simulink model "TH_P_Inv"  (R2023a)
settings: Solver=ode23  StartTime=0.0  StopTime=0.1  RelTol=1e-3
libraries: spsIGBTDiodeLib x6, simulink x3, spsSeriesRLCBranchLib x3, spsDCVoltageSourceLib x1, spsGroundLib x1, spsThreePhaseVIMeasurementLib x1, sps_lib x1

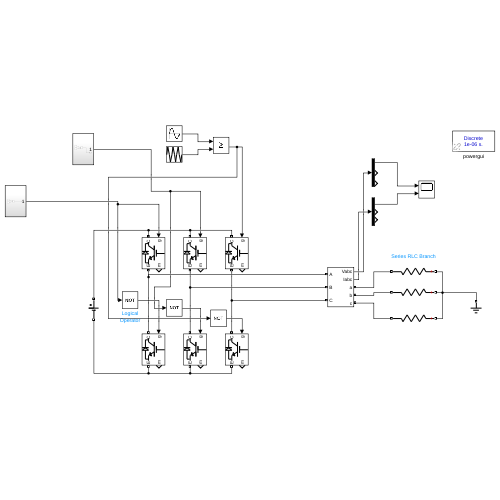
[thumbnail: Simulink's stored preview of the top-level diagram]
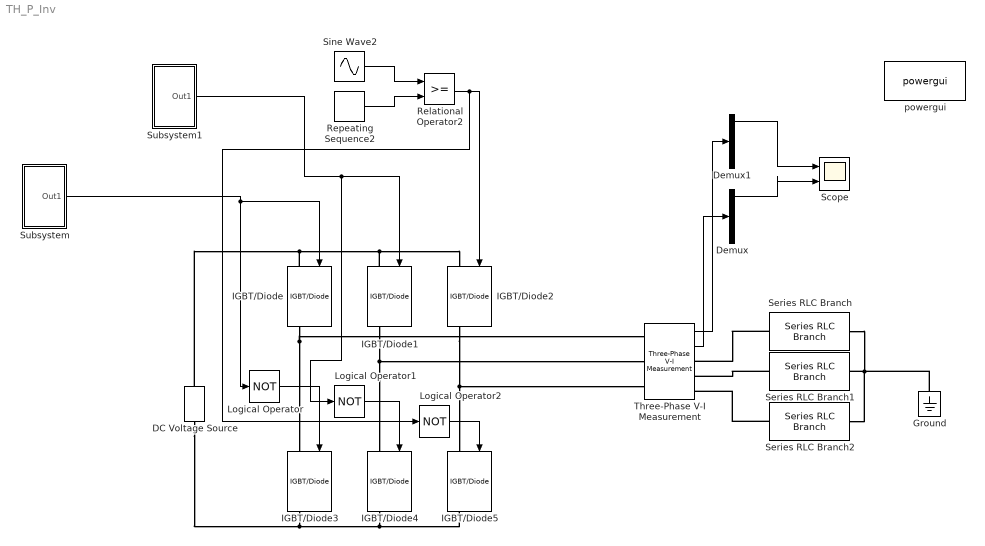
== system TH_P_Inv ==
  DC Voltage Source : spsDCVoltageSourceLib/DC Voltage Source  Amplitude=650  Measurements=None
  Demux : Demux  Outputs=3
  Demux1 : Demux  Outputs=3
  Ground : spsGroundLib/Ground  LConnTagsString=a
  IGBT/Diode{,1..5} (6 alike) : spsIGBTDiodeLib/IGBT//Diode  Ron=1e-3  Rs=1e5  Cs=inf  Measurements=on
  Logical Operator : Logic  Operator=NOT  AllPortsSameDT=off  OutDataTypeStr=boolean
  Logical Operator1 : Logic  Operator=NOT  AllPortsSameDT=off  OutDataTypeStr=boolean
  Logical Operator2 : Logic  Operator=NOT  AllPortsSameDT=off  OutDataTypeStr=boolean
  Relational Operator2 : RelationalOperator  OutDataTypeStr=boolean  RndMeth=Simplest  InputSameDT=off
  Repeating Sequence2 : simulink/Sources/Repeating Sequence  rep_seq_t=[0 0.25/5000 0.5/5000 0.75/5000 1/5000]  rep_seq_y=[0 1 0 -1 0 ]
  Scope : Scope  NumInputPorts=2
  Series RLC Branch : spsSeriesRLCBranchLib/Series RLC Branch  LConnTagsString=__new0  RConnTagsString=__new0  BranchType=R  Resistance=10  Inductance=1e-3  SetiL0=off  InitialCurrent=0  Capacitance=1e-6  Setx0=off  InitialVoltage=0  Measurements=None
  Series RLC Branch1 : spsSeriesRLCBranchLib/Series RLC Branch  LConnTagsString=__new0  RConnTagsString=__new0  BranchType=R  Resistance=10  Inductance=1e-3  SetiL0=off  InitialCurrent=0  Capacitance=1e-6  Setx0=off  InitialVoltage=0  Measurements=None
  Series RLC Branch2 : spsSeriesRLCBranchLib/Series RLC Branch  LConnTagsString=__new0  RConnTagsString=__new0  BranchType=R  Resistance=10  Inductance=1e-3  SetiL0=off  InitialCurrent=0  Capacitance=1e-6  Setx0=off  InitialVoltage=0  Measurements=None
  Sine Wave2 : Sin  Amplitude=0.99  Frequency=100*pi  Phase=(4*pi)/3  SampleTime=0
  Subsystem : Subsystem
  Subsystem1 : Subsystem
  Three-Phase V-I Measurement : spsThreePhaseVIMeasurementLib/Three-Phase V-I Measurement  VoltageMeasurement=phase-to-ground  SetLabelV=off  LabelV=Vabc  Vpu=off  VpuLL=off  CurrentMeasurement=yes  SetLabelI=off  LabelI=Iabc  Ipu=off  Pbase=100e6  Vbase=500e3  OutputType=Complex  PhasorSimulation=off  PSBequivalent=0
  powergui : sps_lib/powergui  Priority=1  SimulationMode=Discrete  SampleTime=1e-6  frequency=60  Iterations=50  frequencyindice=0  Pbase=100e6  ErrMax=1e-4  UnitsV=kV  UnitsW=MW  buscounter=0  FunctionMessages=off  echomessages=off  EnableUseOfTLC=off  CurrentSourceSwitches=off  DisableSnubberDevices=off  DisableRonSwitches=off  DisableVfSwitches=off  DisplayEquations=off  AutomaticDiscreteSolvers=off  SolverType=Tustin/Backward Euler (TBE)  Interpol=off  ExternalGateDelay=off  methode=off  Ts=100  x0status=blocks  SPID=on  SwTol=0  HookPort=off  NonlinearTolerance=1e-4  nMaxIteration=100  ContinueOnMaxIteration=off  RestoreLinks=warning  ResistiveCurrentMeasurement=off  Frange=[0:2:500]  Ylog=off  Xlog=on  ShowGrid=off  save=off  variable=ZData  structure=0  ZoomFFT=off  StartTime=0.0  cycles=1  DisplayStyle=1  fundamental=60  FreqAxis=off  MaxFrequency=1000  frequencyindicesteady=1  RmsSteady=1  display=off
  wires:
  Sine Wave2/1 -> Relational Operator2/1
  Repeating Sequence2/1 -> Relational Operator2/2
  Relational Operator2/1 -> Logical Operator2/1, IGBT/Diode2/1
  Logical Operator/1 -> IGBT/Diode3/1
  Logical Operator2/1 -> IGBT/Diode5/1
  Logical Operator1/1 -> IGBT/Diode4/1
  Three-Phase V-I Measurement/1 -> Demux1/1
  Three-Phase V-I Measurement/2 -> Demux/1
  Demux1/1 -> Scope/1
  Demux/1 -> Scope/2
  Subsystem/1(Out1) -> Logical Operator/1, IGBT/Diode/1
  Subsystem1/1(Out1) -> Logical Operator1/1, IGBT/Diode1/1
  connections:
  DC Voltage Source/RConn1 -- IGBT/Diode/LConn1 -- IGBT/Diode1/LConn1 -- IGBT/Diode2/LConn1
  DC Voltage Source/LConn1 -- IGBT/Diode3/RConn1 -- IGBT/Diode4/RConn1 -- IGBT/Diode5/RConn1
  IGBT/Diode/RConn1 -- IGBT/Diode3/LConn1 -- Three-Phase V-I Measurement/LConn1
  IGBT/Diode1/RConn1 -- IGBT/Diode4/LConn1 -- Three-Phase V-I Measurement/LConn2
  IGBT/Diode2/RConn1 -- IGBT/Diode5/LConn1 -- Three-Phase V-I Measurement/LConn3
  Series RLC Branch/LConn1 -- Ground/LConn1 -- Series RLC Branch2/LConn1 -- Series RLC Branch1/LConn1
  Series RLC Branch/RConn1 -- Three-Phase V-I Measurement/RConn1
  Series RLC Branch1/RConn1 -- Three-Phase V-I Measurement/RConn2
  Series RLC Branch2/RConn1 -- Three-Phase V-I Measurement/RConn3

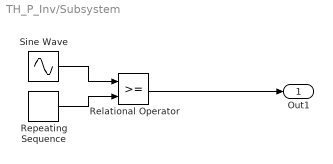
== system TH_P_Inv/Subsystem ==
  Relational Operator : RelationalOperator  OutDataTypeStr=boolean  RndMeth=Simplest  InputSameDT=off
  Repeating Sequence : simulink/Sources/Repeating Sequence  rep_seq_t=[0 0.25/5000 0.5/5000 0.75/5000 1/5000]  rep_seq_y=[0 1 0 -1 0 ]
  Sine Wave : Sin  Amplitude=0.99  Frequency=100*pi  SampleTime=0
  Out1 : Outport
  wires:
  Sine Wave/1 -> Relational Operator/1
  Repeating Sequence/1 -> Relational Operator/2
  Relational Operator/1 -> Out1/1

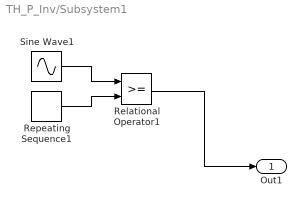
== system TH_P_Inv/Subsystem1 ==
  Relational Operator1 : RelationalOperator  OutDataTypeStr=boolean  RndMeth=Simplest  InputSameDT=off
  Repeating Sequence1 : simulink/Sources/Repeating Sequence  rep_seq_t=[0 0.25/5000 0.5/5000 0.75/5000 1/5000]  rep_seq_y=[0 1 0 -1 0 ]
  Sine Wave1 : Sin  Amplitude=0.99  Frequency=100*pi  Phase=(2*pi)/3  SampleTime=0
  Out1 : Outport
  wires:
  Sine Wave1/1 -> Relational Operator1/1
  Repeating Sequence1/1 -> Relational Operator1/2
  Relational Operator1/1 -> Out1/1
